simulink model "Lenkung_CarMaker_DSR"  (Simulink 7.9)
settings: Solver=ode45  StartTime=0.0  StopTime=20  FixedStep=0.002  RelTol=1e-3
undefined symbols (not defined in the file or in its folder): pin
libraries: simulink x4, cstblocks x3, library x3
settings Model: Creator=Georg  LastModifiedBy=georgnestlinger
settings DebuggingCC: SolverPrmCheckMsg=none  FcnCallInpInsideContextMsg=Use local settings  StrictBusMsg=Warning
settings GRTTargetCC: CombineOutputUpdateFcns=off  GRTInterface=on

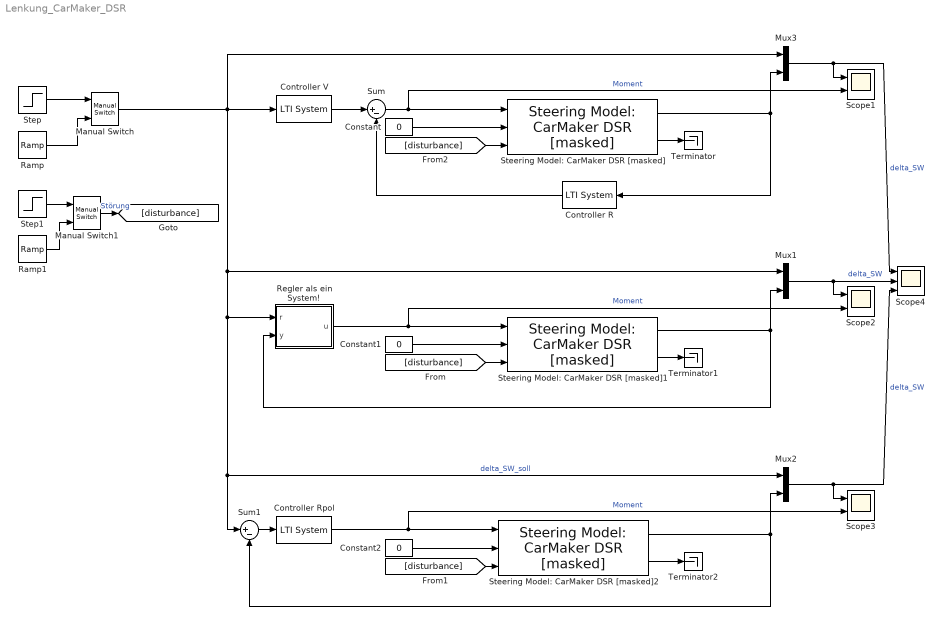
== system Lenkung_CarMaker_DSR ==
  Constant : Constant  Value=0
  Constant1 : Constant  Value=0
  Constant2 : Constant  Value=0
  Controller R : cstblocks/LTI System  sys=R  IC=[]
  Controller Rpol : cstblocks/LTI System  sys=Rpol  IC=[]
  Controller V : cstblocks/LTI System  sys=V  IC=[]
  Manual Switch : simulink/Signal Routing/Manual Switch  sw=1  action=0  varsize=off
  Manual Switch1 : simulink/Signal Routing/Manual Switch  sw=1  action=0  varsize=off
  Mux1 : Mux  Inputs=2
  Mux2 : Mux  Inputs=2
  Mux3 : Mux  Inputs=2
  Ramp : simulink/Sources/Ramp  slope=1  start=10  X0=0
  Ramp1 : simulink/Sources/Ramp  slope=100  start=15  X0=0
  Regler als ein System! : Subsystem
  Scope1 : Scope  NumInputPorts=2
      settings: YMin=-5~-5  YMax=5~5
  Scope2 : Scope  NumInputPorts=2
      settings: YMin=-5~-5  YMax=5~5
  Scope3 : Scope  NumInputPorts=2
      settings: YMin=-5~-5  YMax=5~5  SaveName=ScopeData2
  Scope4 : Scope  NumInputPorts=3
      settings: YMin=-5~-5~-5  YMax=5~5~5  SaveName=ScopeData3
  Steering Model: CarMaker DSR [masked] : library/Steering Models/Steering Model: CarMaker DSR [masked]  d_rot=pin.SteeringModel.parameter.values.drot  d_rack=pin.SteeringModel.parameter.values.drack  i=pin.SteeringModel.parameter.values.iHR  I_rot=pin.SteeringModel.parameter.values.J  m_left=pin.SteeringModel.parameter.values.mL  m_right=pin.SteeringModel.parameter.values.mR  m_rack=pin.SteeringModel.parameter.values.mr  V=pin.SteeringModel.parameter.values.V
  Steering Model: CarMaker DSR [masked]1 : library/Steering Models/Steering Model: CarMaker DSR [masked]  d_rot=pin.SteeringModel.parameter.values.drot  d_rack=pin.SteeringModel.parameter.values.drack  i=pin.SteeringModel.parameter.values.iHR  I_rot=pin.SteeringModel.parameter.values.J  m_left=pin.SteeringModel.parameter.values.mL  m_right=pin.SteeringModel.parameter.values.mR  m_rack=pin.SteeringModel.parameter.values.mr  V=pin.SteeringModel.parameter.values.V
  Steering Model: CarMaker DSR [masked]2 : library/Steering Models/Steering Model: CarMaker DSR [masked]  d_rot=pin.SteeringModel.parameter.values.drot  d_rack=pin.SteeringModel.parameter.values.drack  i=pin.SteeringModel.parameter.values.iHR  I_rot=pin.SteeringModel.parameter.values.J  m_left=pin.SteeringModel.parameter.values.mL  m_right=pin.SteeringModel.parameter.values.mR  m_rack=pin.SteeringModel.parameter.values.mr  V=pin.SteeringModel.parameter.values.V
  Step : Step  SampleTime=0
  Step1 : Step  Time=5  After=100  SampleTime=0
  Sum : Sum  Inputs=|+-
  Sum1 : Sum  Inputs=|+-
  Terminator : Terminator
  Terminator1 : Terminator
  Terminator2 : Terminator
  wires:
  Sum/1 -> Scope1/2, Steering Model: CarMaker DSR [masked]/1  "Moment"
  Mux3/1 -> Scope1/1, Scope4/1  "delta_SW"
  Regler als ein System!/1(u) -> Scope2/2, Steering Model: CarMaker DSR [masked]1/1  "Moment"
  Steering Model: CarMaker DSR [masked]1/1 -> Regler als ein System!/2(y), Mux1/2
  Mux1/1 -> Scope2/1, Scope4/2  "delta_SW"
  Step/1 -> Manual Switch/1
  Ramp/1 -> Manual Switch/2
  Sum1/1 -> Controller Rpol/1
  Steering Model: CarMaker DSR [masked]2/1 -> Sum1/2, Mux2/2
  Mux2/1 -> Scope3/1, Scope4/3  "delta_SW"
  Controller Rpol/1 -> Scope3/2, Steering Model: CarMaker DSR [masked]2/1  "Moment"
  Controller R/1 -> Sum/2
  Controller V/1 -> Sum/1
  Step1/1 -> Manual Switch1/1
  Ramp1/1 -> Manual Switch1/2
  Constant/1 -> Steering Model: CarMaker DSR [masked]/2
  Constant1/1 -> Steering Model: CarMaker DSR [masked]1/2
  Constant2/1 -> Steering Model: CarMaker DSR [masked]2/2
  Manual Switch/1 -> Controller V/1, Mux3/1, Regler als ein System!/1(r), Sum1/1, Mux2/1, Mux1/1  "delta_SW_soll"
  Manual Switch1/1 -> [disturbance]  "Störung"
  [disturbance] -> Steering Model: CarMaker DSR [masked]1/3
  [disturbance] -> Steering Model: CarMaker DSR [masked]2/3
  [disturbance] -> Steering Model: CarMaker DSR [masked]/3
  Steering Model: CarMaker DSR [masked]/1 -> Mux3/2, Controller R/1
  Steering Model: CarMaker DSR [masked]/2 -> Terminator/1
  Steering Model: CarMaker DSR [masked]1/2 -> Terminator1/1
  Steering Model: CarMaker DSR [masked]2/2 -> Terminator2/1

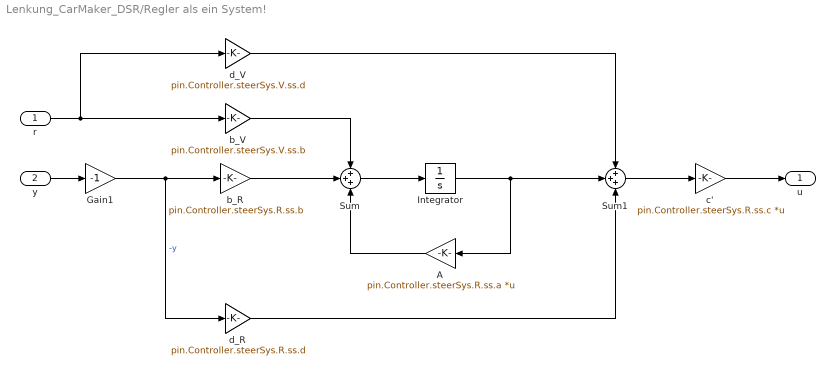
== system Lenkung_CarMaker_DSR/Regler als ein System! ==
  r : Inport
  y : Inport  Port=2
  A : Gain  Gain=pin.Controller.steerSys.R.ss.a  Multiplication=Matrix(K*u)
  Gain1 : Gain  Gain=-1
  Integrator : Integrator  InitialCondition=pin.Controller.steerSys.initialValue
  Sum : Sum  Inputs=+++
  Sum1 : Sum  Inputs=+++
  b_R : Gain  Gain=pin.Controller.steerSys.R.ss.b
  b_V : Gain  Gain=pin.Controller.steerSys.V.ss.b
  c' : Gain  Gain=pin.Controller.steerSys.R.ss.c  Multiplication=Matrix(K*u)
  d_R : Gain  Gain=pin.Controller.steerSys.R.ss.d
  d_V : Gain  Gain=pin.Controller.steerSys.V.ss.d
  u : Outport
  wires:
  Sum1/1 -> c'/1
  d_R/1 -> Sum1/3
  d_V/1 -> Sum1/1
  Integrator/1 -> Sum1/2, A/1
  b_V/1 -> Sum/1
  r/1 -> d_V/1, b_V/1
  b_R/1 -> Sum/2
  Gain1/1 -> d_R/1, b_R/1  "-y"
  y/1 -> Gain1/1
  Sum/1 -> Integrator/1
  A/1 -> Sum/3
  c'/1 -> u/1
